simulink model "Part1"  (R2024b)
settings: Solver=ode4  StartTime=0.0  StopTime=T_SIM  FixedStep=T_s  RelTol=1e-3
values from neighbouring files (symbols this model uses):
  d = d_id    (= 0.18428)    [analysis_data3.m]
  omega_max = 10    [analysis_data3.m]
  r = r_id    (= 0.03316)    [analysis_data3.m]
  T_s = 0.04    [analysis_data3.m]
undefined symbols (not defined in the file or in its folder): D, H, P_INIT_EKF, PHI_INIT, Q_INIT_LOC, R, R_2, R_4, Ta, Tc, Ts, w, X, Y, Z_INIT_EKF
libraries: robotlib x11, sharedtransform x1
settings Model: Creator=tomailoren  LastModifiedBy=loren
settings OptimizationCC: DefaultParameterBehavior=Inlined  EnhancedBackFolding=on  PassReuseOutputArgsAs=Individual arguments  ZeroExternalMemoryAtStartup=off  ZeroInternalMemoryAtStartup=off  MaxStackSize=64  OptimizeBlockOrder=speed  DifferentSizesBufferReuse=on  OptimizationCustomize=off  EfficientTunableParamExpr=on
settings DebuggingCC: ParameterTunabilityLossMsg=error
settings HardwareCC: ProdBitPerPointer=32  ProdBitPerSizeT=32  ProdBitPerPtrDiffT=32  ProdLargestAtomicFloat=None  ProdIntDivRoundTo=Undefined  ProdEndianess=Unspecified  ProdWordSize=32  ProdHWDeviceType=Generic->Unspecified (assume 32-bit Generic)
settings SFSimCC: MATLABDynamicMemAlloc=off
settings RTWCC: Description=Embedded Coder  SystemTargetFile=ert.tlc  HardwareBoard=Robot Operating System (ROS)  TLCOptions="-aInlineSetEventsForThisBaseRateFcn=TLC_FALSE -aSuppressMultiTaskScheduler=TLC_FALSE  -aRateBasedStepFcn=0"  TemplateMakefile=ert_default_tmf  Toolchain=Catkin  TargetLang=C++
settings CodeAppCC: ForceParamTrailComments=on  IgnoreCustomStorageClasses=off  OperatorAnnotations=on  SimulinkDataObjDesc=on  SFDataObjDesc=on  InsertBlockDesc=on

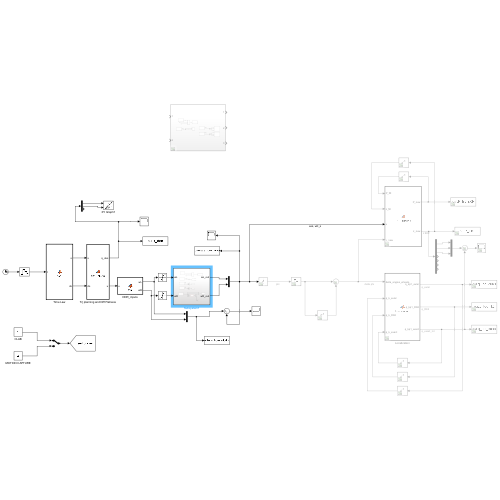
[thumbnail: Simulink's stored preview of the top-level diagram]
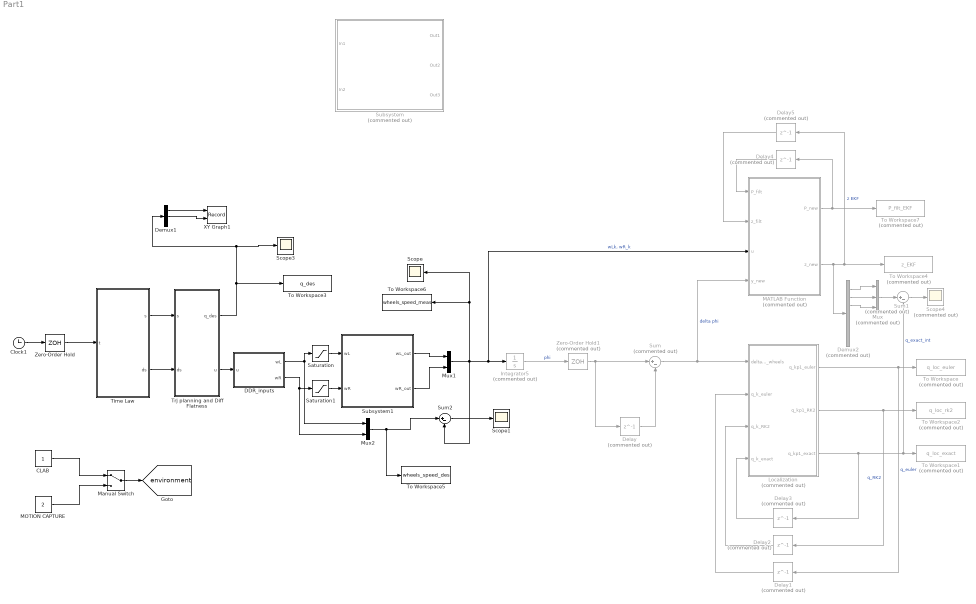
== system Part1 ==
  CLAB : Constant
  Clock1 : Clock
      settings: Decimation=1/T_s
  DDR_inputs : MATLAB Function  TreatAsAtomicUnit=on
  Delay : Delay  Commented=on  DelayLength=1  InitialCondition=[0;0]  SampleTime=T_s
  Delay1 : Delay  Commented=on  DelayLength=1  InitialCondition=Q_INIT_LOC
  Delay2 : Delay  Commented=on  DelayLength=1  InitialCondition=Q_INIT_LOC
  Delay3 : Delay  Commented=on  DelayLength=1  InitialCondition=Q_INIT_LOC
  Delay4 : Delay  Commented=on  DelayLength=1  InitialCondition=P_INIT_EKF  SampleTime=T_s
  Delay5 : Delay  Commented=on  DelayLength=1  InitialCondition=Z_INIT_EKF  SampleTime=T_s
  Demux1 : Demux  Outputs=3
  Demux2 : Demux  Commented=on  Outputs=7
  Integrator5 : Integrator  Commented=on  InitialCondition=PHI_INIT
  Localization : MATLAB Function  Commented=on  TreatAsAtomicUnit=on
  MATLAB Function : MATLAB Function  Commented=on  TreatAsAtomicUnit=on
  MOTION CAPTURE : Constant  Value=2
  Manual Switch : ManualSwitch
  Mux : Mux  Commented=on  Inputs=3
  Mux1 : Mux  Inputs=2
  Mux2 : Mux  Inputs=2
  Saturation : Saturate  UpperLimit=omega_max  LowerLimit=-omega_max
  Saturation1 : Saturate  UpperLimit=omega_max  LowerLimit=-omega_max
  Scope : Scope
  Scope1 : Scope
  Scope3 : Scope
  Scope4 : Scope  Commented=on
  Subsystem : Subsystem  Commented=on
  Subsystem1 : Subsystem
  Sum : Sum  Commented=on  Inputs=|+-
  Sum1 : Sum  Commented=on  Inputs=|+-
  Sum2 : Sum  Inputs=|+-
  Time Law : MATLAB Function  TreatAsAtomicUnit=on
  To Workspace : ToWorkspace  Commented=on  VariableName=q_loc_euler  SaveFormat=Structure With Time  SampleTime=-1
  To Workspace1 : ToWorkspace  Commented=on  VariableName=q_loc_exact  SaveFormat=Structure With Time  SampleTime=-1
  To Workspace2 : ToWorkspace  Commented=on  VariableName=q_loc_rk2  SaveFormat=Structure With Time  SampleTime=-1
  To Workspace3 : ToWorkspace  VariableName=q_des  SaveFormat=Structure With Time  SampleTime=-1
  To Workspace4 : ToWorkspace  Commented=on  VariableName=z_EKF  SaveFormat=Structure With Time  SampleTime=-1
  To Workspace5 : ToWorkspace  VariableName=wheels_speed_des  SaveFormat=Structure With Time  SampleTime=-1
  To Workspace6 : ToWorkspace  VariableName=wheels_speed_meas  SaveFormat=Structure With Time  SampleTime=-1
  To Workspace7 : ToWorkspace  Commented=on  VariableName=P_filt_EKF  SaveFormat=Structure With Time  SampleTime=-1
  Trj planning and Diff Flatness : MATLAB Function  TreatAsAtomicUnit=on
  XY Graph1 : Record  FileSettingsInternal="{\"entries\":[{\"content\":{\"excelSettings\":{\"content\":{},\"type\":\"Streamout.ExcelSettings\"}},\"type\":\"Streamout.FileSettingStorage\",\"uuid\":\"\"}],\"packageUris\":[\"http:\\/\\/schema.mathworks.com\\/mf0\\/streamout_blocks\\/R2020a\"],\"version\":\"1.0\"}"  Layout=[1 1]  SignalsInternal="{\"entries\":[{\"content\":{\"signals\":[{\"content\":{\"blockPath\":[],\"dimensions\":[1,1],\"domain\":\"\",\"lineColor\":\"#a2142f\",\"plots\":[ 1 ],\"port\":1,\"signalID\":1,\"signalName\":\"Demux1:1\"},\"type\":\"RecordBlkView.Signal\",\"uuid\":\"\"},{\"content\":{\"blockPath\":[],\"dimensions\":[1,1],\"domain\":\"\",\"lineColor\":\"#139fff\",\"plots\":[ 1 ],\"port\":2,\"signalID\":2,\"signalName\":\"Demux1:2\"},\"type\":\"RecordBlkView.Signal\",\"uuid\":\"\"}]},\"type\":\"RecordBlkView.InputSignals\",\"uuid\":\"\"}],\"packageUris\":[\"http:\\/\\/schema.mathworks.com\\/mf0\\/streamout_blocks\\/R2020a\"],\"version\":\"1.0\"}"  VisualizationBindings="{\"xyplotplugin\":{\"info\":[{\"series\":[{\"bindingParametersList\":[{\"parameter\":\"X-Axis\",\"signalID\":1,\"signalName\":\"Demux1:1\"},{\"parameter\":\"Y-Axis\",\"signalID\":2,\"signalName\":\"Demux1:2\"}],\"seriesID\":0}],\"subplotID\":1}]}}"  CompatibilityTag=XY
  Zero-Order Hold : ZeroOrderHold  SampleTime=T_s
  Zero-Order Hold1 : ZeroOrderHold  Commented=on  SampleTime=T_s
  tag scope: environment=global
  wires:
  Demux1/1 -> XY Graph1/1
  MATLAB Function/2(z_new) -> Demux2/1, To Workspace4/1, Delay5/1  "z EKF"
  Time Law/1(s) -> Trj planning and Diff Flatness/1(s)
  Mux1/1 -> Integrator5/1, MATLAB Function/3(u), Sum2/2, Scope/1, To Workspace6/1  "wLk, wR_k"
  Delay1/1 -> Localization/2(q_k_euler)
  Zero-Order Hold/1 -> Time Law/1(t)
  Demux2/2 -> Mux/2
  Trj planning and Diff Flatness/1(q_des) -> To Workspace3/1, Scope3/1, Demux1/1
  Zero-Order Hold1/1 -> Sum/1, Delay/1
  Clock1/1 -> Zero-Order Hold/1
  Demux2/3 -> Mux/3
  Delay5/1 -> MATLAB Function/2(z_filt)
  Delay/1 -> Sum/2
  Delay3/1 -> Localization/4(q_k_exact)
  Integrator5/1 -> Zero-Order Hold1/1  "phi"
  Localization/2(q_kp1_RK2) -> To Workspace2/1, Delay2/1  "q_RK2"
  Localization/1(q_kp1_euler) -> To Workspace/1, Delay1/1  "q_euler"
  Time Law/2(ds) -> Trj planning and Diff Flatness/2(ds)
  Delay2/1 -> Localization/3(q_k_RK2)
  Sum1/1 -> Scope4/1
  Mux/1 -> Sum1/1
  Trj planning and Diff Flatness/2(u) -> DDR_inputs/1(u)
  Sum/1 -> MATLAB Function/4(y_new), Localization/1(delta_angles_wheels)  "delta phi"
  Delay4/1 -> MATLAB Function/1(P_filt)
  Localization/3(q_kp1_exact) -> To Workspace1/1, Sum1/2, Delay3/1  "q_exact_int"
  Demux2/1 -> Mux/1
  MATLAB Function/1(P_new) -> To Workspace7/1, Delay4/1
  Demux1/2 -> XY Graph1/2
  Subsystem1/1(wL_out) -> Mux1/1
  Subsystem1/2(wR_out) -> Mux1/2
  DDR_inputs/1(wL) -> Saturation/1, Mux2/1
  Saturation/1 -> Subsystem1/1(wL)
  DDR_inputs/2(wR) -> Mux2/2, Saturation1/1
  Saturation1/1 -> Subsystem1/2(wR)
  Mux2/1 -> To Workspace5/1, Sum2/1
  Sum2/1 -> Scope1/1
  CLAB/1 -> Manual Switch/1
  MOTION CAPTURE/1 -> Manual Switch/2
  Manual Switch/1 -> [environment]

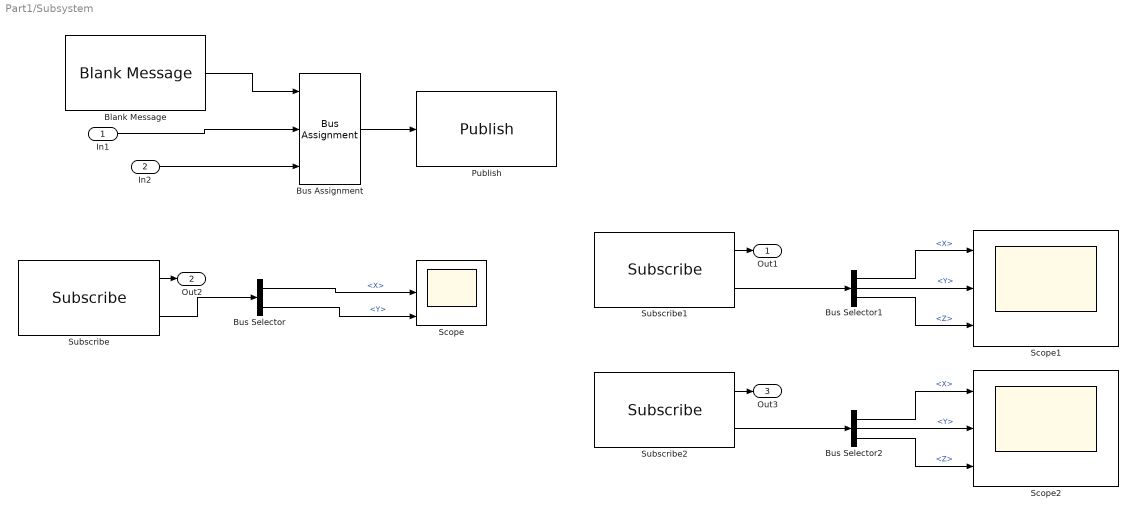
== system Part1/Subsystem ==
  In1 : Inport
  In2 : Inport  Port=2
  Blank Message : robotlib/Blank Message  messageClass=Message  entityType=geometry_msgs/Vector3  messageType=geometry_msgs/Vector3  SampleTime=Ts  legacyBusStruct=off
  Bus Assignment : BusAssignment  AssignedSignals=X,Y
  Bus Selector : BusSelector  OutputSignals=X,Y
  Bus Selector1 : BusSelector  OutputSignals=X,Y,Z
  Bus Selector2 : BusSelector  OutputSignals=X,Y,Z
  Publish : robotlib/Publish  topicSource=Select from ROS network  topic=/turtlebot_01/cmd_wheels  messageType=geometry_msgs/Vector3  legacyBusStruct=off  messageQueueLength=1
  Scope : Scope  NumInputPorts=3
  Scope1 : Scope  NumInputPorts=3
  Scope2 : Scope  NumInputPorts=3
  Subscribe : robotlib/Subscribe  topicSource=Select from ROS network  topic=/turtlebot_01/wheelSpeeds  messageType=geometry_msgs/Vector3  SampleTime=Ts  legacyBusStruct=off  messageQueueLength=1
  Subscribe1 : robotlib/Subscribe  topicSource=Select from ROS network  topic=/turtlebot_01/gyroscope  messageType=geometry_msgs/Vector3  SampleTime=Ts  legacyBusStruct=off  messageQueueLength=1
  Subscribe2 : robotlib/Subscribe  topicSource=Select from ROS network  topic=/turtlebot_01/accelerometer  messageType=geometry_msgs/Vector3  SampleTime=Ts  legacyBusStruct=off  messageQueueLength=1
  Out1 : Outport
  Out2 : Outport  Port=2
  Out3 : Outport  Port=3
  wires:
  Bus Selector1/2 -> Scope1/2  "<Y>"
  Subscribe/2 -> Bus Selector/1
  Bus Selector2/1 -> Scope2/1  "<X>"
  Bus Selector1/3 -> Scope1/3  "<Z>"
  Bus Selector2/2 -> Scope2/2  "<Y>"
  Subscribe1/1 -> Out1/1
  Bus Assignment/1 -> Publish/1
  Bus Selector1/1 -> Scope1/1  "<X>"
  Bus Selector/1 -> Scope/2  "<X>"
  In2/1 -> Bus Assignment/3
  Subscribe1/2 -> Bus Selector1/1
  Subscribe2/2 -> Bus Selector2/1
  Blank Message/1 -> Bus Assignment/1
  Bus Selector/2 -> Scope/3  "<Y>"
  Bus Selector2/3 -> Scope2/3  "<Z>"
  In1/1 -> Bus Assignment/2
  Subscribe2/1 -> Out3/1
  Subscribe/1 -> Out2/1

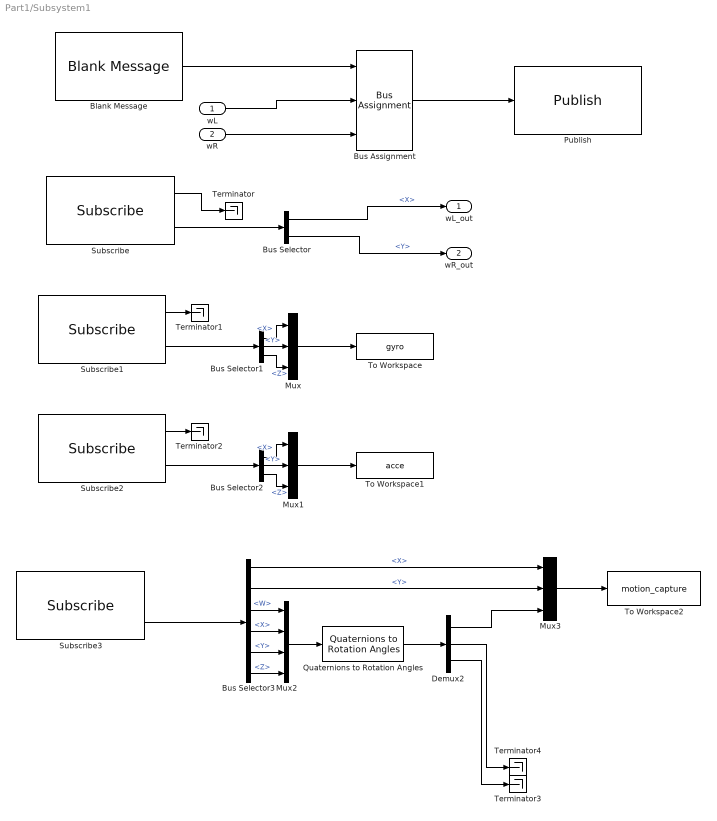
== system Part1/Subsystem1 ==
  wL : Inport
  wR : Inport  Port=2
  Blank Message : robotlib/Blank Message  messageClass=Message  entityType=geometry_msgs/Vector3  messageType=geometry_msgs/Vector3  SampleTime=T_s  legacyBusStruct=off
  Bus Assignment : BusAssignment  AssignedSignals=X,Y
  Bus Selector : BusSelector  OutputSignals=X,Y
  Bus Selector1 : BusSelector  OutputSignals=X,Y,Z
  Bus Selector2 : BusSelector  OutputSignals=X,Y,Z
  Bus Selector3 : BusSelector  OutputSignals=Pose.Pose.Position.X,Pose.Pose.Position.Y,Pose.Pose.Orientation.W,Pose.Pose.Orientation.X,Pose.Pose.Orientation.Y,Pose.Pose.Orientation.Z
  Demux2 : Demux  Outputs=3
  Mux : Mux  Inputs=3
  Mux1 : Mux  Inputs=3
  Mux2 : Mux
  Mux3 : Mux  Inputs=3
  Publish : robotlib/Publish  topicSource=Select from ROS network  topic=/turtlebot_01/cmd_wheels  messageType=geometry_msgs/Vector3  legacyBusStruct=off  messageQueueLength=1
  Quaternions to Rotation Angles : sharedtransform/Quaternions to Rotation Angles  rotationOrder=ZYX  aMode=aMode
  Subscribe : robotlib/Subscribe  topicSource=Select from ROS network  topic=/turtlebot_01/wheelSpeeds  messageType=geometry_msgs/Vector3  SampleTime=T_s  legacyBusStruct=off  messageQueueLength=1
  Subscribe1 : robotlib/Subscribe  topicSource=Select from ROS network  topic=/turtlebot_01/gyroscope  messageType=geometry_msgs/Vector3  SampleTime=T_s  legacyBusStruct=off  messageQueueLength=1
  Subscribe2 : robotlib/Subscribe  topicSource=Select from ROS network  topic=/turtlebot_01/accelerometer  messageType=geometry_msgs/Vector3  SampleTime=T_s  legacyBusStruct=off  messageQueueLength=1
  Subscribe3 : robotlib/Subscribe  topicSource=Select from ROS network  topic=/turtlebot_01/odom  messageType=nav_msgs/Odometry  SampleTime=T_s  legacyBusStruct=off  messageQueueLength=1
      settings: LibrarySourceBlock=roslib/ROS/Subscribe
  Terminator{,1..4} (5 alike) : Terminator
  To Workspace : ToWorkspace  VariableName=gyro  SaveFormat=Structure With Time  SampleTime=-1
  To Workspace1 : ToWorkspace  VariableName=acce  SaveFormat=Structure With Time  SampleTime=-1
  To Workspace2 : ToWorkspace  VariableName=motion_capture  SaveFormat=Structure With Time  SampleTime=-1
  wL_out : Outport
  wR_out : Outport  Port=2
  wires:
  wL/1 -> Bus Assignment/2
  Bus Assignment/1 -> Publish/1
  wR/1 -> Bus Assignment/3
  Blank Message/1 -> Bus Assignment/1
  Subscribe/1 -> Terminator/1
  Bus Selector/1 -> wL_out/1  "<X>"
  Subscribe/2 -> Bus Selector/1
  Bus Selector/2 -> wR_out/1  "<Y>"
  Subscribe1/1 -> Terminator1/1
  Subscribe2/1 -> Terminator2/1
  Subscribe1/2 -> Bus Selector1/1
  Subscribe2/2 -> Bus Selector2/1
  Bus Selector1/1 -> Mux/1  "<X>"
  Bus Selector1/2 -> Mux/2  "<Y>"
  Bus Selector1/3 -> Mux/3  "<Z>"
  Bus Selector2/1 -> Mux1/1  "<X>"
  Bus Selector2/2 -> Mux1/2  "<Y>"
  Bus Selector2/3 -> Mux1/3  "<Z>"
  Mux/1 -> To Workspace/1
  Mux1/1 -> To Workspace1/1
  Quaternions to Rotation Angles/1 -> Demux2/1
  Demux2/1 -> Mux3/3
  Bus Selector3/6 -> Mux2/4  "<Z>"
  Bus Selector3/5 -> Mux2/3  "<Y>"
  Demux2/3 -> Terminator3/1
  Bus Selector3/4 -> Mux2/2  "<X>"
  Bus Selector3/2 -> Mux3/2  "<Y>"
  Bus Selector3/1 -> Mux3/1  "<X>"
  Subscribe3/2 -> Bus Selector3/1
  Bus Selector3/3 -> Mux2/1  "<W>"
  Demux2/2 -> Terminator4/1
  Mux2/1 -> Quaternions to Rotation Angles/1
  Mux3/1 -> To Workspace2/1

== matlab function Part1/Time Law ==
  data: t input; s output; ds output; Ta parameter; Tc parameter
function [s, ds] = fcn(t, Ta, Tc)
          
    vc = 1/(Ta+Tc);
    a = vc/Ta;
   
    if t < Ta
        s_dot = a*t;
        s = 0.5*a*t^2;
    
    elseif t < (Ta+Tc)
        s_dot = vc;
        s = 0.5*a*Ta^2 + vc*(t - Ta);
    
    elseif t < (2*Ta+Tc)
        s_dot = vc - a*(t - Ta - Tc);
        s = 0.5*a*Ta^2 + vc*Tc + vc*(t - Ta - Tc) ...
            - 0.5*a*(t - Ta - Tc)^2;
    else
        s_dot = 0;
        s = 1;
    end

    ds = s_dot;
    
end

== matlab function Part1/Trj planning and Diff Flatness ==
  data: q_des output; s input; u output; ds input; R parameter; w parameter
function [q_des, u] = get_inputs(s, ds, R, w)

    % function [x_s, y_s, x_s_dot, y_s_dot, x_s_ddot, y_s_ddot] = gen_eight_shape_trajectory(R, w, s)
   
    x_s = R*sin(2*w*s);
    y_s = R*sin(w*s);
    
    % computes derivatives analytically

    x_s_dot = 2*R*w*cos(2*w*s);
    y_s_dot = R*w*cos(w*s);
    
    x_s_ddot = -4*R*w^2*sin(2*w*s);
    y_s_ddot = -R*w^2*sin(w*s);


    % function [q, u] = flat_to_kinematic_cartesian(x, y, x_dot, y_dot, x_ddot, y_ddot)

    theta = atan2(y_s_dot, x_s_dot);
    
    q_des = [x_s; y_s; theta];
   
    v_tilde = sqrt(x_s_dot^2 + y_s_dot^2);
    omega_tilde = (x_s_dot * y_s_ddot - y_s_dot * x_s_ddot) / (x_s_dot^2 + y_s_dot^2);
    
    % Convert into real Inputs
    v = v_tilde * ds;
    omega = omega_tilde * ds;
    
    u = [v; omega];
end

== matlab function Part1/Localization ==
  data: delta_angles_wheels input; q_k_euler input; q_k_RK2 input; q_k_exact input; r parameter; d parameter; q_kp1_euler output; T_s parameter; q_kp1_RK2 output; q_kp1_exact output
function [q_kp1_euler, q_kp1_RK2, q_kp1_exact] = localization(delta_angles_wheels, q_k_euler, q_k_RK2, q_k_exact, r, d, T_s)

    % extraction data
    delta_phi_L = delta_angles_wheels(1);
    delta_phi_R = delta_angles_wheels(2);

    x_k_euler = q_k_euler(1); 
    y_k_euler = q_k_euler(2); 
    theta_k_euler = q_k_euler(3);
    
    x_k_RK2 = q_k_RK2(1); 
    y_k_RK2 = q_k_RK2(2); 
    theta_k_RK2 = q_k_RK2(3);

    x_k_exact = q_k_exact(1);
    y_k_exact = q_k_exact(2); 
    theta_k_exact = q_k_exact(3);


    % velocities estimate
    v_k = r / (2*T_s) * (delta_phi_R + delta_phi_L);
    w_k = r / (d*T_s) * (delta_phi_R - delta_phi_L);
    
    % Euler integration
    x_kp1_euler = x_k_euler + v_k * T_s * cos(theta_k_euler);
    y_kp1_euler = y_k_euler + v_k * T_s * sin(theta_k_euler);
    theta_kp1_euler = theta_k_euler + w_k * T_s;
    
    q_kp1_euler = [x_kp1_euler; y_kp1_euler; theta_kp1_euler];
    
    % RK2 Integration
    x_kp1_RK2 = x_k_RK2 + v_k * T_s * cos(theta_k_RK2 + (w_k * T_s)/2);
    y_kp1_RK2 = y_k_RK2 + v_k * T_s * sin(theta_k_RK2 + (w_k * T_s)/2);
    theta_kp1_RK2 = theta_k_RK2 + w_k * T_s;
    
    q_kp1_RK2 = [x_kp1_RK2; y_kp1_RK2; theta_kp1_RK2];
    
    % Exact Integration
    if abs(w_k) < 1e-4
        % use RK2 approximation to avoid division by zero when w_k is near 0
        x_kp1_exact = x_k_exact + v_k * T_s * cos(theta_k_exact + (w_k * T_s)/2);
        y_kp1_exact = y_k_exact + v_k * T_s * sin(theta_k_exact + (w_k * T_s)/2);
    else
        % Exact formulas
        x_kp1_exact = x_k_exact + (v_k / w_k) * (sin(theta_k_exact + w_k * T_s) - sin(theta_k_exact));
        y_kp1_exact = y_k_exact - (v_k / w_k) * (cos(theta_k_exact + w_k * T_s) - cos(theta_k_exact));
    end
    theta_kp1_exact = theta_k_exact + w_k * T_s;
    
    q_kp1_exact = [x_kp1_exact; y_kp1_exact; theta_kp1_exact];
    
end

== matlab function Part1/MATLAB Function ==
  data: P_filt input; P_new output; z_filt input; z_new output; u input; y_new input; D parameter; R_2 parameter; R_4 parameter; T_s parameter; r parameter; d parameter; H parameter
function [P_new, z_new] = EKF_filtering(P_filt, z_filt, u, y_new, D, R_2, R_4, T_s, r, d,H)

    % Def state z_filt: [xk , yk , thetak , delta_phi_L_km1 , delta_phi_R_km1 , wLk , wRk ]
    
    % Extraction variables
    x_k = z_filt(1);
    y_k = z_filt(2);
    theta_k = z_filt(3);
    delta_phi_L_km1 = z_filt(4);
    delta_phi_R_km1 = z_filt(5); 
    wL_k = z_filt(6);               % estimate wheels velocities
    wR_k = z_filt(7);
    
    uL_k = u(1);                    % actual wheels velocities (from command input v,w)
    uR_k = u(2);

    % ----------------------

    % PREDICT STEP
    v_k = (r/2) * (wL_k + wR_k);
    omega_k = (r/d) * (wR_k - wL_k);
    theta_mean = theta_k + (omega_k * T_s) / 2;
        
    % State Prediction (approximation with RK2)
    x_kp1 = x_k + v_k * T_s * cos(theta_mean);
    y_kp1 = y_k + v_k * T_s * sin(theta_mean);
    theta_kp1 = theta_k + omega_k * T_s;
    
    delta_phi_L_k = wL_k * T_s;
    delta_phi_R_k = wR_k * T_s;
    
    wL_kp1 = uL_k; 
    wR_kp1 = uR_k;
    
    z_hat = [x_kp1; y_kp1; theta_kp1; delta_phi_L_k; delta_phi_R_k; wL_kp1; wR_kp1];
    
    % F derivation
    F = zeros(7,7);
    
    F(1,1) = 1;
    F(1, 3) = -T_s * v_k * sin(theta_mean);
    F(1, 6) = (T_s * r / 2) * cos(theta_mean) - v_k * T_s * sin(theta_mean) * (-T_s * r / (2 * d));
    F(1, 7) = (T_s * r / 2) * cos(theta_mean) - v_k * T_s * sin(theta_mean) * (T_s * r / (2 * d));
    
    F(2,2) = 1;
    F(2, 3) = v_k * T_s * cos(theta_mean);
    F(2, 6) = (T_s * r / 2) * sin(theta_mean) + v_k * T_s * cos(theta_mean) * (-T_s * r / (2 * d));
    F(2, 7) = (T_s * r / 2) * sin(theta_mean) + v_k * T_s * cos(theta_mean) * (T_s * r / (2 * d));

    F(3,3) = 1;
    F(3, 6) = -T_s * r / d;
    F(3, 7) = T_s * r / d;

    F(4, 6) = T_s;
    F(5, 7) = T_s;
    
    % Covariance Prediction
    P_hat = F * P_filt * F' + D;
    
    % ----------------------

    % UPDATE STEP
   
    % Observation Matrix H 
    % H1: delta angles sensor (delta_phi_L, delta_phi_R)
    %H = [0, 0, 0, 1, 0, 0, 0;
         %0, 0, 0, 0, 1, 0, 0];

    % Innovation e_pred
    y_hat = H * z_hat;
    e_kp1 = y_new - y_hat;
    
    % Kalman Gain K_pred
    K = P_hat * H' / ( H * P_hat * H' + R_2 );   
    
    % State and Covariance Update
    z_new = z_hat + K * e_kp1;
    P_new = P_hat - K * H * P_hat;

end

== matlab function Part1/DDR_inputs ==
  data: u input; wL output; wR output; r parameter; d parameter
function [wL, wR] = fcn(u,r, d)

    v = u(1);
    omega = u(2);

    wL = v/r - (d*omega)/(2*r);
    wR = v/r + (d*omega)/(2*r);

end
